simulink model "steam_generator"  (R2021a)
settings: Solver=VariableStepAuto  StartTime=0.0  StopTime=10  RelTol=1e-3
values from neighbouring files (symbols this model uses):
  err_weights = 0.3    [full_plant_20.m]    (also in sg.m = 0.5)
  h_fw = h_sg_out0 - P_thermal0 * 1e3 / num_sg / W_o0    [full_plant.m]    (also in full_plant_20.m; policy.m = h_sg_out0 - P_thermal0 * 1e3 / num_sg / W0; reactor_core.m = h_sg_out0 - P_thermal0 * 1e3 / num_sg / W0; sg.m = h_sg_out0 - P_thermal0 * 1e3 / num_sg / W0)
  M_sg = P_thermal0 / (T_h0 - T_c0) / num_sg    (= 46.3537906137)    [full_plant.m]    (also in full_plant_20.m; policy.m; reactor_core.m; sg.m)
  mu_m = 8.46    [full_plant.m]    (also in full_plant_20.m; policy.m; reactor_core.m; sg.m)
  mu_p = 141.0    (= 141)    [full_plant.m]    (also in full_plant_20.m; policy.m; reactor_core.m; sg.m)
  P_sg0 = 6.38    [full_plant.m]    (also in full_plant_20.m; policy.m; reactor_core.m; sg.m)
  T_h0 = 317.7    [full_plant.m]    (also in full_plant_20.m; policy.m; reactor_core.m; sg.m)
  T_m0 = (T_p0 + T_sg_out0) / 2    [full_plant.m]    (also in full_plant_20.m = (T_c0 + T_sg_out0) / 2; policy.m; reactor_core.m; sg.m)
  T_p0 = (T_h0 + T_c0) / 2    (= 303.85)    [full_plant.m]    (also in policy.m; reactor_core.m; sg.m)
  V_f0 = 74.94    [full_plant.m]    (also in full_plant_20.m; policy.m; reactor_core.m; sg.m)
  V_sg = 259.92    [full_plant.m]    (also in full_plant_20.m; policy.m; reactor_core.m; sg.m)
  W_fw0 = 680.4    [full_plant.m]    (also in full_plant_20.m)
  W_o0 = 680.4    [full_plant.m]    (also in full_plant_20.m)
  Z1 = P_thermal0 / (T_p0 - T_m0) / num_sg    [full_plant.m]    (also in full_plant_20.m = P_thermal0 / (T_c0 - T_m0) / num_sg; policy.m; reactor_core.m; sg.m)
  Z2 = P_thermal0 / (T_m0 - T_sg_out0) / num_sg    [full_plant.m]    (also in full_plant_20.m; policy.m; reactor_core.m; sg.m)
settings Model: Creator=xxc90  LastModifiedBy=xxc90

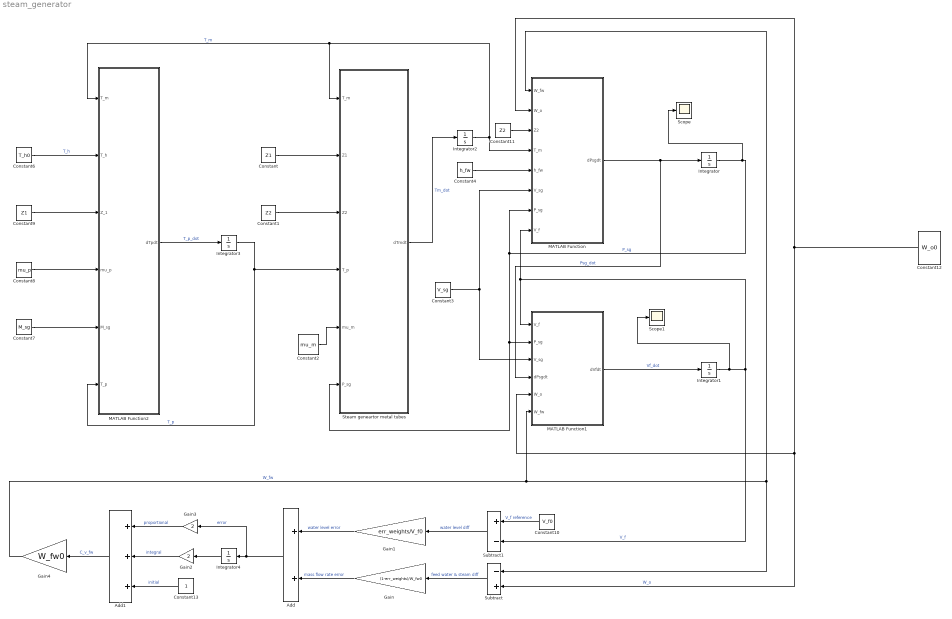
== system steam_generator ==
  Add : Sum
  Add1 : Sum  Inputs=+++
  Constant : Constant  Value=Z1
  Constant1 : Constant  Value=Z2
  Constant10 : Constant  Value=V_f0
  Constant11 : Constant  Value=Z2
  Constant12 : Constant  Value=W_o0
  Constant13 : Constant
  Constant2 : Constant  Value=mu_m
  Constant3 : Constant  Value=V_sg
  Constant4 : Constant  Value=h_fw
  Constant6 : Constant  Value=T_h0
  Constant7 : Constant  Value=M_sg
  Constant8 : Constant  Value=mu_p
  Constant9 : Constant  Value=Z1
  Gain : Gain  Gain=(1-err_weights)/W_fw0
  Gain1 : Gain  Gain=err_weights/V_f0
  Gain2 : Gain  Gain=2
  Gain3 : Gain  Gain=2
  Gain4 : Gain  Gain=W_fw0
  Integrator : Integrator  InitialCondition=P_sg0
  Integrator1 : Integrator  InitialCondition=V_f0
  Integrator2 : Integrator  InitialCondition=T_m0
  Integrator3 : Integrator  InitialCondition=T_p0
  Integrator4 : Integrator
  MATLAB Function : MATLAB Function  TreatAsAtomicUnit=on
  MATLAB Function1 : MATLAB Function  TreatAsAtomicUnit=on
  MATLAB Function2 : MATLAB Function  TreatAsAtomicUnit=on
  Scope : Scope
  Scope1 : Scope
  Steam geneartor metal tubes : MATLAB Function  TreatAsAtomicUnit=on
  Subtract : Sum  Inputs=-+
  Subtract1 : Sum  Inputs=+-
  wires:
  MATLAB Function/1(dPsgdt) -> MATLAB Function1/4(dPsgdt), Integrator/1  "Psg_dot"
  Integrator/1 -> Scope/1, Steam geneartor metal tubes/6(P_sg), MATLAB Function1/2(P_sg), MATLAB Function/7(P_sg)  "P_sg"
  MATLAB Function1/1(dVfdt) -> Integrator1/1  "Vf_dot"
  Integrator1/1 -> Scope1/1, Subtract1/2, MATLAB Function1/1(V_f), MATLAB Function/8(V_f)  "V_f"
  Steam geneartor metal tubes/1(dTmdt) -> Integrator2/1  "Tm_dot"
  Integrator2/1 -> Steam geneartor metal tubes/1(T_m), MATLAB Function2/1(T_m), MATLAB Function/4(T_m)  "T_m"
  Integrator3/1 -> Steam geneartor metal tubes/4(T_p), MATLAB Function2/6(T_p)  "T_p"
  Constant/1 -> Steam geneartor metal tubes/2(Z1)
  Constant1/1 -> Steam geneartor metal tubes/3(Z2)
  Constant2/1 -> Steam geneartor metal tubes/5(mu_m)
  Constant3/1 -> MATLAB Function1/3(V_sg), MATLAB Function/6(V_sg)
  Constant4/1 -> MATLAB Function/5(h_fw)
  Constant6/1 -> MATLAB Function2/2(T_h)  "T_h"
  Constant7/1 -> MATLAB Function2/5(M_sg)
  Constant8/1 -> MATLAB Function2/4(mu_p)
  Constant9/1 -> MATLAB Function2/3(Z_1)
  MATLAB Function2/1(dTpdt) -> Integrator3/1  "T_p_dot"
  Constant11/1 -> MATLAB Function/3(Z2)
  Gain4/1 -> MATLAB Function1/6(W_fw), Subtract/1, MATLAB Function/1(W_fw)  "W_fw"
  Constant12/1 -> Subtract/2, MATLAB Function1/5(W_o), MATLAB Function/2(W_o)  "W_o"
  Subtract/1 -> Gain/1  "feed water & steam diff"
  Constant10/1 -> Subtract1/1  "V_f reference"
  Subtract1/1 -> Gain1/1  "water level diff"
  Gain1/1 -> Add/1  "water level error"
  Gain/1 -> Add/2  "mass flow rate error"
  Add/1 -> Gain3/1, Integrator4/1  "error"
  Integrator4/1 -> Gain2/1
  Gain3/1 -> Add1/1  "proportional"
  Gain2/1 -> Add1/2  "integral"
  Constant13/1 -> Add1/3  "initial"
  Add1/1 -> Gain4/1  "C_v_fw"

== matlab function steam_generator/MATLAB Function1 ==
  data: V_f input; P_sg input; V_sg input; dPsgdt input; W_o input; W_fw input; dVfdt output
function dVfdt = dVfdt(V_f, P_sg, V_sg, dPsgdt, W_o, W_fw)
    rho_f = XSteam('rhoL_p', P_sg*10);
    rho_g = XSteam('rhoV_p', P_sg*10);
    dP = 0.01;
    drhogdP = (XSteam('rhoV_p', P_sg*10+ dP) - XSteam('rhoV_p', P_sg*10)) / dP;
    dVfdt = (W_fw - W_o - (V_sg - V_f)* drhogdP * dPsgdt) / (rho_f - rho_g);
end

== matlab function steam_generator/MATLAB Function ==
  data: W_fw input; dPsgdt output; W_o input; Z2 input; T_m input; h_fw input; V_sg input; P_sg input; V_f input
function dPsgdt= dPsgdt(W_fw, W_o, Z2, T_m, h_fw, V_sg, P_sg, V_f)
    T_s = XSteam('Tsat_p', P_sg*10);
    rho_g = XSteam('rhoV_p', P_sg*10);
    u_g = XSteam('uV_p', P_sg*10);
    h_g = XSteam('hV_p', P_sg*10)
    rho_f = XSteam('rhoL_p', P_sg*10);
    u_f = XSteam('uL_p', P_sg*10);
    dP = 0.01;
    dufdP = (XSteam('uL_p', P_sg*10+ dP) - XSteam('uL_p', P_sg*10)) / dP;
    dugdP = (XSteam('uV_p', P_sg*10+ dP) - XSteam('uV_p', P_sg*10)) / dP;
    drhofdP = (XSteam('rhoL_p', P_sg*10+ dP) - XSteam('rhoL_p', P_sg*10)) / dP;
    drhogdP = (XSteam('rhoV_p', P_sg*10+ dP) - XSteam('rhoV_p', P_sg*10)) / dP;
    dPsgdt_num = W_fw * h_fw - W_o * h_g + Z2 * (T_m - T_s) * 1000 + (rho_g*u_g - rho_f*u_f)/(rho_f-rho_g)*(W_fw - W_o);
    dPsgdt_den = rho_f * V_f * dufdP + (V_sg - V_f) * u_g * drhogdP + rho_g * (V_sg - V_f) * dugdP + (V_sg - V_f) * (rho_g*u_g - rho_f*u_f)/(rho_f-rho_g) * drhogdP ;
    dPsgdt = dPsgdt_num / dPsgdt_den;
end

== matlab function steam_generator/Steam geneartor metal tubes ==
  data: T_m input; dTmdt output; Z1 input; Z2 input; T_p input; mu_m input; P_sg input
function dTmdt = dTmdt(T_m, Z1, Z2, T_p, mu_m, P_sg)
    T_s = XSteam('Tsat_p', P_sg*10);
    dTmdt = (Z1 * (T_p - T_m) - Z2*(T_m - T_s)) / mu_m
end

== matlab function steam_generator/MATLAB Function2 ==
  data: T_m input; T_h input; Z_1 input; mu_p input; M_sg input; dTpdt output; T_p input
function dTpdt = dTpdt(T_m, T_h, Z_1, mu_p, M_sg, T_p)
    T_c = 2 * T_p - T_h
    dTpdt = (M_sg * (T_h - T_c) - Z_1 * (T_p - T_m)) / mu_p
end
